simulink model "acdcac_simscape"  (R2014a)
settings: Solver=ode23t  StartTime=0.0  StopTime=0.2  RelTol=1e-3
PreLoadFcn:
  | Ts = 2e-6;
  | Tc = 5e-4;
InitFcn:
  | Ts = 2e-6;
  | Tc = 5e-4;
StartFcn:
  | tic;
StopFcn:
  | toc;
undefined symbols (not defined in the file): DiscIntNeverNeededParam
libraries: pe_lib x11, nesl_utility x11, fl_lib x9, powerlib_meascontrol x3, simulink x2
settings Model: Creator=skadetot  LastModifiedBy=cosorio
settings SolverCC: MaxConsecutiveZCs=5000
settings DataIOCC: LimitDataPoints=off  SaveOutput=off  SaveTime=off  SignalLoggingName=sigsOutSC
settings DebuggingCC: UnderspecifiedInitializationDetection=Classic  SolverPrmCheckMsg=none

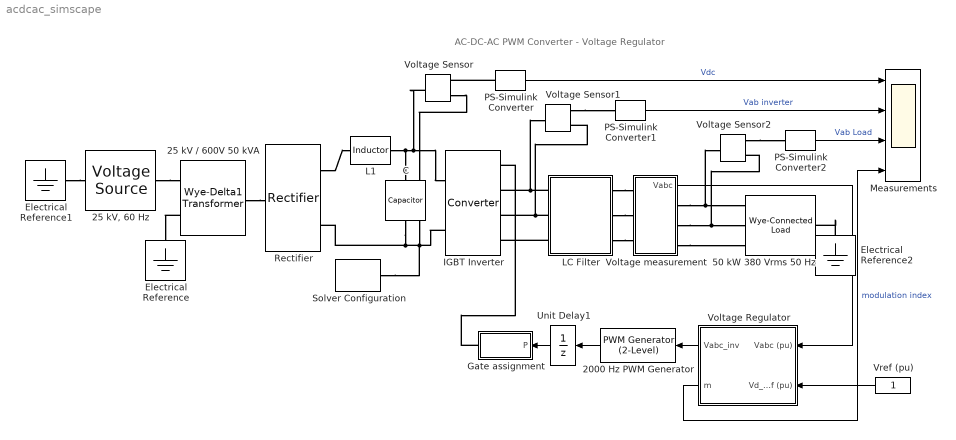
== system acdcac_simscape ==
  note: AC-DC-AC PWM Converter - Voltage Regulator
  2000 Hz PWM Generator : powerlib_meascontrol/Pulse & Signal Generators/PWM Generator (2-Level)  ModulatorType=Three-phase bridge (6 pulses)  ModulatorMode=Unsynchronized  nF=27  Fc=2000  ModulatingSignals=off  m=0.8  Freq=60  Phase=0  Ts=Ts
  25 kV / 600V 50 kVA : pe_lib/Passive Devices/Transformers/Wye-Delta1 Transformer  SRated=50e3/sqrt(3) V*A  VRated1=25e3/sqrt(3) V  VRated2=600 V  FRated=60 Hz  pu_Rl1=0.004  pu_Xl1=0.02  pu_Rl2=0.004  pu_Xl2=0.02  pu_Rm=200  pu_Xm=200  i1_0=[0, 0, 0] A  i2_0=[0, 0, 0] A  im0=[0, 0, 0] A  phi0=[0, 0, 0] Wb  Rl1=nan Ohm  Ll1=nan H  Rl2=nan Ohm  Ll2=nan H  Rm=nan Ohm  Lm=nan H
  "25 kV, 60 Hz" : pe_lib/Sources/Voltage Source  vline_rms=25e3 V  shift=0 deg  freq=60 Hz  omega=0 rad/s  shift_3ph=[nan, nan, nan]  sqrt2OverSqrt3=nan
  50 kW 380 Vrms 50 Hz : pe_lib/Passive Devices/Wye-Connected Load  parameterization=2  component_structure=1  component_structure_PQ=1  R=1 Ohm  L=0.001 H  C=1e-6 F  IL0=[ 0 0 0 ] A  VC0=[ 0 0 0 ] V  R_parasitic=1e-6 Ohm  G_parasitic=1e-6 1/Ohm  VRated=380 V  FRated=60 Hz  P=50e3 W  Qpos=100 V*A  Qneg=-100 V*A  Vmag0=2.4e+4 V  Vang0=0 deg  Freq0=60 Hz  R_parasitic_PQ=1e-6 Ohm  G_parasitic_PQ=1e-6 1/Ohm
  C : fl_lib/Electrical/Electrical Elements/Capacitor  c=5000e-6 F  r=1e-6 Ohm  g=0 1/Ohm  i_specify=off  i_priority=High  i=0 A  v_specify=off  v_priority=High  v=0 V  vc_specify=on  vc_priority=High  vc=0 V
  Electrical Reference : fl_lib/Electrical/Electrical Elements/Electrical Reference
  Electrical Reference1 : fl_lib/Electrical/Electrical Elements/Electrical Reference
  Electrical Reference2 : fl_lib/Electrical/Electrical Elements/Electrical Reference
  Gate assignment : Subsystem
  IGBT Inverter : pe_lib/Semiconductors/Converter  device_type=3  Vf=0.001 V  Ron=0.001 Ohm  Rds=0.001 Ohm  Goff=1e-6 1/Ohm  Vth=0.5 V  Vgt=1 V  Vgt_off=-1 V  Ih=1 A  diode_param=2  diode_Vf=0.8 V  diode_Ron=0.001 Ohm  diode_Goff=1e-6 1/Ohm  diode_C=50 nF  diode_iRM=-235 A  diode_iF=300 A  diode_idot=-50 A/us  diode_trr_param=1  diode_trr_factor=3  diode_trr=15 us  diode_Qrr=1.5e+3 s*uA  snubber_type=0  Rs=0.1 Ohm  Cs=1e-7 F
  L1 : fl_lib/Electrical/Electrical Elements/Inductor  l=200e-6 H  r=0 Ohm  g=1e-9 1/Ohm  i_specify=off  i_priority=High  i=0 A  v_specify=off  v_priority=High  v=0 V  i_L_specify=on  i_L_priority=High  i_L=0 A
  LC Filter : Subsystem
  Measurements : Scope  NumInputPorts=4
      settings: YMin=0~-1000~-600~0  YMax=1200~1000~600~1.2  SaveName=ACDCACSimscape
  PS-Simulink Converter : nesl_utility/PS-Simulink Converter  PhysicalDomain=network_engine_domain  SubClassName=ps_output  LeftPortType=input  RightPortType=output  PseudoPeriodic=off  Frequencies=[]  Unit=V  AffineConversion=off
  PS-Simulink Converter1 : nesl_utility/PS-Simulink Converter  PhysicalDomain=network_engine_domain  SubClassName=ps_output  LeftPortType=input  RightPortType=output  PseudoPeriodic=off  Frequencies=[]  Unit=V  AffineConversion=off
  PS-Simulink Converter2 : nesl_utility/PS-Simulink Converter  PhysicalDomain=network_engine_domain  SubClassName=ps_output  LeftPortType=input  RightPortType=output  PseudoPeriodic=off  Frequencies=[]  Unit=V  AffineConversion=off
  Rectifier : pe_lib/Semiconductors/Rectifier  model_dynamics=0  Vf=0.8 V  Ron=0.01 Ohm  Goff=1e-6 1/Ohm  C=50 nF  iRM=-235 A  iF=300 A  idot=-50 A/us  trr_param=1  trr_factor=3  trr=15 us  Qrr=1.5e+3 s*uA
  Solver Configuration : nesl_utility/Solver Configuration  PhysicalDomain=network_engine_domain  SubClassName=solver  LeftPortType=input  RightPortType=generic  Accelerate=off  Tones=[]  Harmonics=[]  SimulateNoise=off  Profile=off  UseLocalSampling=off  EnableSwitchedLinearOptims=on  FrequencyDomain=off  UseCCode=off  RelTol=0.001  AbsTol=1e-06  MinStep=1e-09  ToWorkspace=off  DoDC=off  ResidualTolerance=1e-09  UseLocalSolver=off  LocalSolverChoice=NE_BACKWARD_EULER_ADVANCER  LocalSolverSampleTime=Ts  DoFixedCost=off  MaxNonlinIter=5  MaxModeIter=2  LinearAlgebra=Sparse  DelaysMemoryBudget=1024  AutomaticFiltering=on  FilteringTimeConstant=0.001
  Unit Delay1 : UnitDelay  SampleTime=Ts
  Voltage Regulator : Subsystem  TreatAsAtomicUnit=on  SystemSampleTime=Tc
  Voltage Sensor : fl_lib/Electrical/Electrical Sensors/Voltage Sensor
  Voltage Sensor1 : fl_lib/Electrical/Electrical Sensors/Voltage Sensor
  Voltage Sensor2 : fl_lib/Electrical/Electrical Sensors/Voltage Sensor
  Voltage measurement : Subsystem
  "Vref (pu) " : Constant  SampleTime=Tc
  wires:
  PS-Simulink Converter/1 -> Measurements/1  "Vdc"
  PS-Simulink Converter1/1 -> Measurements/2  "Vab inverter"
  PS-Simulink Converter2/1 -> Measurements/3  "Vab Load"
  Voltage measurement/1(Vabc) -> Voltage Regulator/1(Vabc (pu))
  "Vref (pu) "/1 -> Voltage Regulator/2(Vd_ref (pu))
  Voltage Regulator/2(m) -> Measurements/4  "modulation index"
  Voltage Regulator/1(Vabc_inv) -> 2000 Hz PWM Generator/1
  2000 Hz PWM Generator/1 -> Unit Delay1/1
  Unit Delay1/1 -> Gate assignment/1(P)
  connections:
  25 kV / 600V 50 kVA/LConn2 -- Electrical Reference/LConn1
  "25 kV, 60 Hz"/RConn1 -- 25 kV / 600V 50 kVA/LConn1
  25 kV / 600V 50 kVA/RConn1 -- Rectifier/LConn1
  Rectifier/RConn1 -- L1/LConn1
  L1/RConn1 -- IGBT Inverter/RConn1 -- Voltage Sensor/LConn1 -- C/LConn1
  IGBT Inverter/RConn2 -- Voltage Sensor/RConn2 -- Solver Configuration/RConn1 -- C/RConn1 -- Rectifier/RConn2
  PS-Simulink Converter/LConn1 -- Voltage Sensor/RConn1
  LC Filter/LConn1 -- Voltage Sensor1/LConn1 -- IGBT Inverter/LConn2
  LC Filter/LConn2 -- Voltage Sensor1/RConn2 -- IGBT Inverter/LConn3
  LC Filter/LConn3 -- IGBT Inverter/LConn4
  Gate assignment/RConn1 -- IGBT Inverter/LConn1
  Electrical Reference1/LConn1 -- "25 kV, 60 Hz"/LConn1
  Voltage Sensor1/RConn1 -- PS-Simulink Converter1/LConn1
  Electrical Reference2/LConn1 -- 50 kW 380 Vrms 50 Hz/RConn1
  Voltage Sensor2/RConn1 -- PS-Simulink Converter2/LConn1
  LC Filter/RConn1 -- Voltage measurement/LConn1
  LC Filter/RConn2 -- Voltage measurement/LConn2
  LC Filter/RConn3 -- Voltage measurement/LConn3
  Voltage measurement/RConn2 -- 50 kW 380 Vrms 50 Hz/LConn2 -- Voltage Sensor2/RConn2
  Voltage measurement/RConn1 -- 50 kW 380 Vrms 50 Hz/LConn1 -- Voltage Sensor2/LConn1
  Voltage measurement/RConn3 -- 50 kW 380 Vrms 50 Hz/LConn3

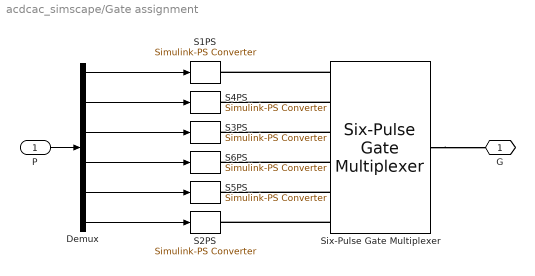
== system acdcac_simscape/Gate assignment ==
  P : Inport
  Demux : Demux  Outputs=6
  S1PS : nesl_utility/Simulink-PS Converter  PhysicalDomain=network_engine_domain  SubClassName=ps_input  LeftPortType=input  RightPortType=output  PseudoPeriodic=off  Frequencies=[]  NoiseDistribution=none  NoiseParameters=[]  Unit=V  AffineConversion=off  InputFiltering=off  SimscapeFilterOrder=1  InputFilterTimeConstant=.001  UdotUserProvided=1
  S2PS : nesl_utility/Simulink-PS Converter  PhysicalDomain=network_engine_domain  SubClassName=ps_input  LeftPortType=input  RightPortType=output  PseudoPeriodic=off  Frequencies=[]  NoiseDistribution=none  NoiseParameters=[]  Unit=V  AffineConversion=off  InputFiltering=off  SimscapeFilterOrder=1  InputFilterTimeConstant=.001  UdotUserProvided=1
  S3PS : nesl_utility/Simulink-PS Converter  PhysicalDomain=network_engine_domain  SubClassName=ps_input  LeftPortType=input  RightPortType=output  PseudoPeriodic=off  Frequencies=[]  NoiseDistribution=none  NoiseParameters=[]  Unit=V  AffineConversion=off  InputFiltering=off  SimscapeFilterOrder=1  InputFilterTimeConstant=.001  UdotUserProvided=1
  S4PS : nesl_utility/Simulink-PS Converter  PhysicalDomain=network_engine_domain  SubClassName=ps_input  LeftPortType=input  RightPortType=output  PseudoPeriodic=off  Frequencies=[]  NoiseDistribution=none  NoiseParameters=[]  Unit=V  AffineConversion=off  InputFiltering=off  SimscapeFilterOrder=1  InputFilterTimeConstant=.001  UdotUserProvided=1
  S5PS : nesl_utility/Simulink-PS Converter  PhysicalDomain=network_engine_domain  SubClassName=ps_input  LeftPortType=input  RightPortType=output  PseudoPeriodic=off  Frequencies=[]  NoiseDistribution=none  NoiseParameters=[]  Unit=V  AffineConversion=off  InputFiltering=off  SimscapeFilterOrder=1  InputFilterTimeConstant=.001  UdotUserProvided=1
  S6PS : nesl_utility/Simulink-PS Converter  PhysicalDomain=network_engine_domain  SubClassName=ps_input  LeftPortType=input  RightPortType=output  PseudoPeriodic=off  Frequencies=[]  NoiseDistribution=none  NoiseParameters=[]  Unit=V  AffineConversion=off  InputFiltering=off  SimscapeFilterOrder=1  InputFilterTimeConstant=.001  UdotUserProvided=1
  Six-Pulse Gate Multiplexer : pe_lib/Semiconductors/Six-Pulse Gate Multiplexer  R=0 Ohm
  G : PMIOPort  Port=1  Side=Right
  wires:
  Demux/6 -> S2PS/1
  Demux/5 -> S5PS/1
  Demux/4 -> S6PS/1
  Demux/3 -> S3PS/1
  Demux/2 -> S4PS/1
  Demux/1 -> S1PS/1
  P/1 -> Demux/1
  connections:
  Six-Pulse Gate Multiplexer/LConn1 -- S1PS/RConn1
  Six-Pulse Gate Multiplexer/LConn2 -- S4PS/RConn1
  Six-Pulse Gate Multiplexer/RConn1 -- G/RConn1
  Six-Pulse Gate Multiplexer/LConn3 -- S3PS/RConn1
  Six-Pulse Gate Multiplexer/LConn6 -- S2PS/RConn1
  Six-Pulse Gate Multiplexer/LConn5 -- S5PS/RConn1
  Six-Pulse Gate Multiplexer/LConn4 -- S6PS/RConn1

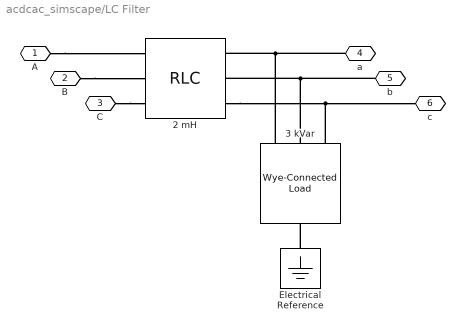
== system acdcac_simscape/LC Filter ==
  2 mH : pe_lib/Passive Devices/RLC  component_structure=2  R=1 Ohm  L=2e-3 H  IL0=[ 0 0 0 ] A  C=1e-6 F  VC0=[ 0 0 0 ] V  R_parasitic=1e-6 Ohm  G_parasitic=1e-6 1/Ohm
  3 kVar : pe_lib/Passive Devices/Wye-Connected Load  parameterization=2  component_structure=3  component_structure_PQ=3  R=1 Ohm  L=0.001 H  C=500e-9 F  IL0=[ 0 0 0 ] A  VC0=[ 0 0 0 ] V  R_parasitic=1e-6 Ohm  G_parasitic=1e-6 1/Ohm  VRated=380 V  FRated=50 Hz  P=1000 W  Qpos=100 V*A  Qneg=-3e3 V*A  Vmag0=380 V  Vang0=0 deg  Freq0=50 Hz  R_parasitic_PQ=1e-6 Ohm  G_parasitic_PQ=1e-6 1/Ohm
  Electrical Reference : fl_lib/Electrical/Electrical Elements/Electrical Reference
  A : PMIOPort  Port=1  Side=Left
  B : PMIOPort  Port=2  Side=Left
  C : PMIOPort  Port=3  Side=Left
  a : PMIOPort  Port=4  Side=Right
  b : PMIOPort  Port=5  Side=Right
  c : PMIOPort  Port=6  Side=Right
  connections:
  Electrical Reference/LConn1 -- 3 kVar/RConn1
  A/RConn1 -- 2 mH/LConn1
  B/RConn1 -- 2 mH/LConn2
  C/RConn1 -- 2 mH/LConn3
  a/RConn1 -- 2 mH/RConn1 -- 3 kVar/LConn1
  b/RConn1 -- 2 mH/RConn2 -- 3 kVar/LConn2
  2 mH/RConn3 -- 3 kVar/LConn3 -- c/RConn1

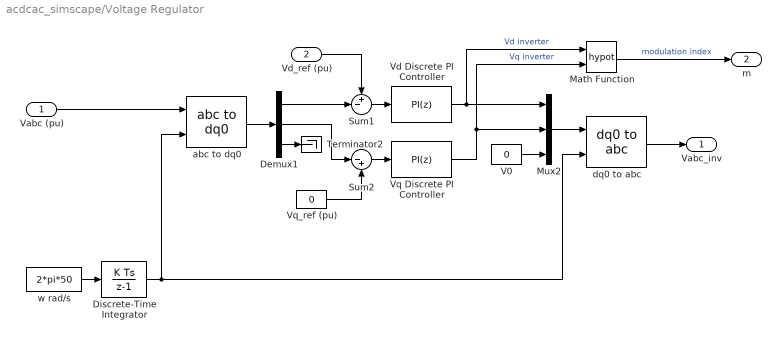
== system acdcac_simscape/Voltage Regulator ==
  Vabc (pu) : Inport
  Vd_ref (pu) : Inport  Port=2
  Demux1 : Demux  Outputs=3
  Discrete-Time Integrator : DiscreteIntegrator  SampleTime=Tc  ICPrevOutput=DiscIntNeverNeededParam  ICPrevScaledInput=DiscIntNeverNeededParam
  Math Function : Math  Operator=hypot  SampleTime=Tc  SaturateOnIntegerOverflow=on
  Mux2 : Mux  Inputs=3
  Sum1 : Sum  Inputs=+-|  SaturateOnIntegerOverflow=on  InputSameDT=on  OutDataTypeStr=Inherit: Same as first input
  Sum2 : Sum  Inputs=|-+  SaturateOnIntegerOverflow=on  InputSameDT=on  OutDataTypeStr=Inherit: Same as first input
  Terminator2 : Terminator
  V0 : Constant  Value=0  SampleTime=Tc
  Vd Discrete PI Controller : simulink/Continuous/PID Controller  Controller=PI  TimeDomain=Discrete-time  SampleTime=Tc  IntegratorMethod=Forward Euler  FilterMethod=Forward Euler  Form=Parallel  P=0.4  I=500  D=0  N=100  InitialConditionSource=internal  InitialConditionForIntegrator=0  InitialConditionForFilter=0  ExternalReset=none  LimitOutput=on  UpperSaturationLimit=1  LowerSaturationLimit=0  LinearizeAsGain=on  AntiWindupMode=none  Kb=1  TrackingMode=off  Kt=1  PParamMin=[]  PParamMax=[]  IParamMin=[]  IParamMax=[]  DParamMin=[]  DParamMax=[]  NParamMin=[]  NParamMax=[]  KbParamMin=[]  KbParamMax=[]  KtParamMin=[]  KtParamMax=[]  POutMin=[]  POutMax=[]  IOutMin=[]  IOutMax=[]  DOutMin=[]  DOutMax=[]  NOutMin=[]  NOutMax=[]  KbOutMin=[]  KbOutMax=[]  KtOutMin=[]  KtOutMax=[]  IntegratorOutMin=[]  IntegratorOutMax=[]  FilterOutMin=[]  FilterOutMax=[]  SumOutMin=[]  SumOutMax=[]  SumI1OutMin=[]  SumI1OutMax=[]  SumI2OutMin=[]  SumI2OutMax=[]  SumI3OutMin=[]  SumI3OutMax=[]  SumDOutMin=[]  SumDOutMax=[]  SaturationOutMin=[]  SaturationOutMax=[]  IntegratorContinuousStateAttributes=''  IntegratorStateMustResolveToSignalObject=off  IntegratorRTWStateStorageClass=Auto  FilterContinuousStateAttributes=''  FilterStateMustResolveToSignalObject=off  FilterRTWStateStorageClass=Auto
  Vq Discrete PI Controller : simulink/Continuous/PID Controller  Controller=PI  TimeDomain=Discrete-time  SampleTime=Tc  IntegratorMethod=Forward Euler  FilterMethod=Forward Euler  Form=Parallel  P=0.4  I=500  D=0  N=100  InitialConditionSource=internal  InitialConditionForIntegrator=0  InitialConditionForFilter=0  ExternalReset=none  LimitOutput=on  UpperSaturationLimit=1  LowerSaturationLimit=0  LinearizeAsGain=on  AntiWindupMode=none  Kb=1  TrackingMode=off  Kt=1  PParamMin=[]  PParamMax=[]  IParamMin=[]  IParamMax=[]  DParamMin=[]  DParamMax=[]  NParamMin=[]  NParamMax=[]  KbParamMin=[]  KbParamMax=[]  KtParamMin=[]  KtParamMax=[]  POutMin=[]  POutMax=[]  IOutMin=[]  IOutMax=[]  DOutMin=[]  DOutMax=[]  NOutMin=[]  NOutMax=[]  KbOutMin=[]  KbOutMax=[]  KtOutMin=[]  KtOutMax=[]  IntegratorOutMin=[]  IntegratorOutMax=[]  FilterOutMin=[]  FilterOutMax=[]  SumOutMin=[]  SumOutMax=[]  SumI1OutMin=[]  SumI1OutMax=[]  SumI2OutMin=[]  SumI2OutMax=[]  SumI3OutMin=[]  SumI3OutMax=[]  SumDOutMin=[]  SumDOutMax=[]  SaturationOutMin=[]  SaturationOutMax=[]  IntegratorContinuousStateAttributes=''  IntegratorStateMustResolveToSignalObject=off  IntegratorRTWStateStorageClass=Auto  FilterContinuousStateAttributes=''  FilterStateMustResolveToSignalObject=off  FilterRTWStateStorageClass=Auto
  Vq_ref (pu) : Constant  Value=0  SampleTime=Tc
  abc to dq0 : powerlib_meascontrol/Transformations/abc to dq0  Alignment=90 degrees behind phase A axis
  dq0 to abc : powerlib_meascontrol/Transformations/dq0 to abc  Alignment=90 degrees behind phase A axis
  w rad/s : Constant  Value=2*pi*50
  Vabc_inv : Outport
  m : Outport  Port=2
  wires:
  Math Function/1 -> m/1  "modulation index"
  Vd Discrete PI Controller/1 -> Mux2/1, Math Function/1  "Vd inverter"
  dq0 to abc/1 -> Vabc_inv/1
  Mux2/1 -> dq0 to abc/1
  Sum1/1 -> Vd Discrete PI Controller/1
  abc to dq0/1 -> Demux1/1
  Sum2/1 -> Vq Discrete PI Controller/1
  Vq_ref (pu)/1 -> Sum2/2
  Demux1/2 -> Sum2/1
  Vq Discrete PI Controller/1 -> Mux2/2, Math Function/2  "Vq inverter"
  V0/1 -> Mux2/3
  Demux1/1 -> Sum1/2
  Vd_ref (pu)/1 -> Sum1/1
  Demux1/3 -> Terminator2/1
  Vabc (pu)/1 -> abc to dq0/1
  Discrete-Time Integrator/1 -> abc to dq0/2, dq0 to abc/2
  w rad/s/1 -> Discrete-Time Integrator/1

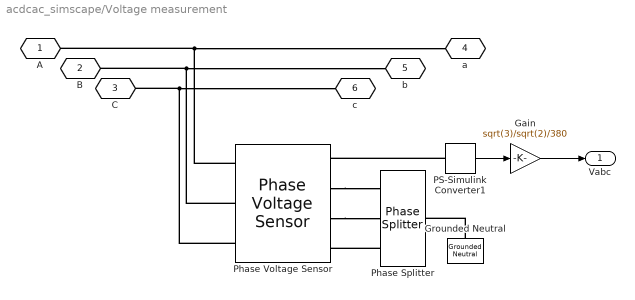
== system acdcac_simscape/Voltage measurement ==
  Gain : Gain  Gain=sqrt(3)/sqrt(2)/380
  Grounded Neutral : pe_lib/Connections/Grounded Neutral
  PS-Simulink Converter1 : nesl_utility/PS-Simulink Converter  PhysicalDomain=network_engine_domain  SubClassName=ps_output  LeftPortType=input  RightPortType=output  PseudoPeriodic=off  Frequencies=[]  Unit=V  AffineConversion=off
  Phase Splitter : pe_lib/Connections/Phase Splitter
  Phase Voltage Sensor : pe_lib/Sensors/Phase Voltage Sensor
  A : PMIOPort  Port=1  Side=Left
  B : PMIOPort  Port=2  Side=Left
  C : PMIOPort  Port=3  Side=Left
  a : PMIOPort  Port=4  Side=Right
  b : PMIOPort  Port=5  Side=Right
  c : PMIOPort  Port=6  Side=Right
  Vabc : Outport
  wires:
  Gain/1 -> Vabc/1
  PS-Simulink Converter1/1 -> Gain/1
  connections:
  PS-Simulink Converter1/LConn1 -- Phase Voltage Sensor/RConn1
  Phase Voltage Sensor/LConn2 -- B/RConn1 -- b/RConn1
  Phase Voltage Sensor/LConn1 -- A/RConn1 -- a/RConn1
  Phase Voltage Sensor/LConn3 -- C/RConn1 -- c/RConn1
  Phase Voltage Sensor/RConn3 -- Phase Splitter/RConn2
  Phase Voltage Sensor/RConn2 -- Phase Splitter/RConn1
  Phase Splitter/RConn3 -- Phase Voltage Sensor/RConn4
  Grounded Neutral/LConn1 -- Phase Splitter/LConn1
